simulink model "IDENTIFICACION_PLATAFORMA_MOVIL_2017"  (R2018b)
settings: Solver=ode3  StartTime=0.0  StopTime=tf  FixedStep=To  RelTol=1e-3  EnableMultiTasking=on
values from neighbouring files (symbols this model uses):
  land = 23.5    [ESTIMACION_PARAMETROS.m]
  To = ts    [ESTIMACION_PARAMETROS.m]
settings Model: Creator=Administrador  LastModifiedBy=lfrec
settings DataIOCC: LimitDataPoints=on  SaveFormat=Array  SignalLoggingSaveFormat=ModelDataLogs
settings OptimizationCC: ExpressionDepthLimit=2147483647  InitFltsAndDblsToZero=on  LifeSpan=inf
settings DebuggingCC: UnderspecifiedInitializationDetection=Classic  MergeDetectMultiDrivingBlocksExec=none  SolverPrmCheckMsg=warning  FcnCallInpInsideContextMsg=warning  StateNameClashWarn=warning  SFUnexpectedBacktrackingDiag=warning  SFNoUnconditionalDefaultTransitionDiag=warning  SFExecutionAtInitializationDiag=none
settings HardwareCC: ProdBitPerPointer=32  ProdBitPerSizeT=32  ProdBitPerPtrDiffT=32  ProdLargestAtomicFloat=None  ProdIntDivRoundTo=Undefined  ProdEndianess=Unspecified  ProdWordSize=32  ProdHWDeviceType=32-bit Generic
settings ModelReferenceCC: PropagateSignalLabelsOutOfModel=off
settings SFSimCC: SimUseLocalCustomCode=off
settings RTWCC: RTWUseLocalCustomCode=off
settings CodeAppCC: StateflowObjectComments=on
settings GRTTargetCC: TargetLangStandard=C89/C90 (ANSI)  CombineOutputUpdateFcns=off  GRTInterface=on
settings ConfigComp: CovMetricSettings=dw  CovHtmlReporting=on  CovSaveCumulativeToWorkspaceVar=on  CovSaveSingleToWorkspaceVar=on  CovExternalEMLEnable=off

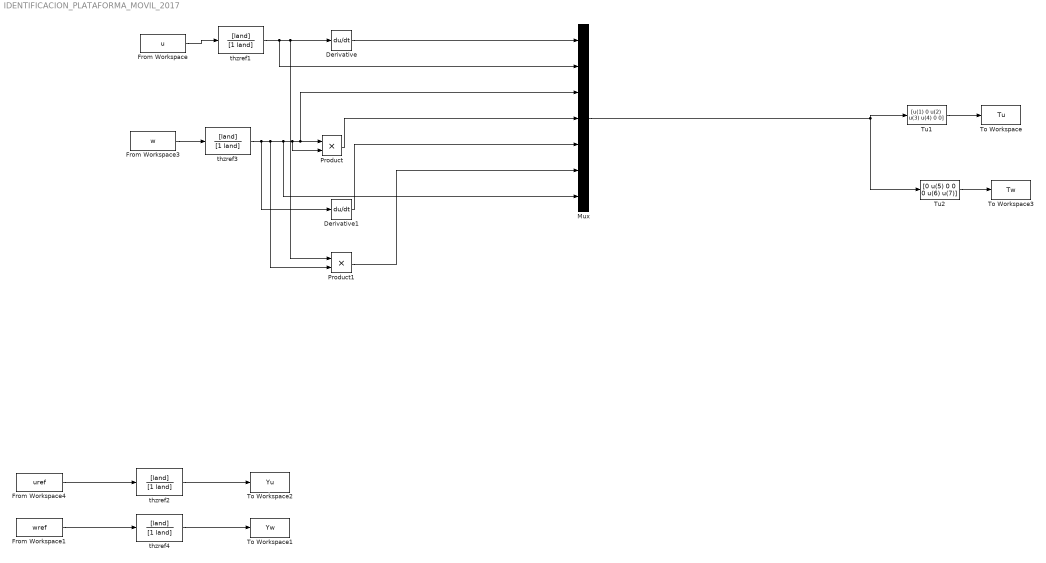
== system IDENTIFICACION_PLATAFORMA_MOVIL_2017 ==
  Derivative : Derivative
  Derivative1 : Derivative
  From Workspace : FromWorkspace  VariableName=u  SampleTime=To
  From Workspace1 : FromWorkspace  VariableName=wref  SampleTime=To
  From Workspace3 : FromWorkspace  VariableName=w  SampleTime=To
  From Workspace4 : FromWorkspace  VariableName=uref  SampleTime=To
  Mux : Mux  Inputs=7
  Product : Product
  Product1 : Product
  To Workspace : ToWorkspace  VariableName=Tu  SampleTime=To
  To Workspace1 : ToWorkspace  VariableName=Yw  SampleTime=To
  To Workspace2 : ToWorkspace  VariableName=Yu  SampleTime=To
  To Workspace3 : ToWorkspace  VariableName=Tw  SampleTime=To
  Tu1 : MATLABFcn  MATLABFcn=[u(1) 0 u(2) u(3) u(4) 0 0]  SampleTime=To
  Tu2 : MATLABFcn  MATLABFcn=[0 u(5) 0 0 0 u(6) u(7)]  SampleTime=To
  thzref{1..4} (4 alike) : TransferFcn  Numerator=[land]  Denominator=[1 land]
  wires:
  From Workspace4/1 -> thzref2/1
  Tu1/1 -> To Workspace/1
  Mux/1 -> Tu1/1, Tu2/1
  From Workspace/1 -> thzref1/1
  thzref2/1 -> To Workspace2/1
  From Workspace1/1 -> thzref4/1
  thzref4/1 -> To Workspace1/1
  Tu2/1 -> To Workspace3/1
  From Workspace3/1 -> thzref3/1
  thzref3/1 -> Derivative1/1, Product1/2, Mux/7, Product/2, Mux/3, Product/1
  Derivative/1 -> Mux/1
  thzref1/1 -> Mux/2, Product1/1, Derivative/1
  Product/1 -> Mux/4
  Derivative1/1 -> Mux/5
  Product1/1 -> Mux/6
